simulink model "p5"  (R2020a)
settings: Solver=VariableStepAuto  StartTime=0.0  StopTime=inf  RelTol=1e-3
undefined symbols (not defined in the file): serial
libraries: instrumentlib x2
settings Model: Creator=escob  LastModifiedBy=escob

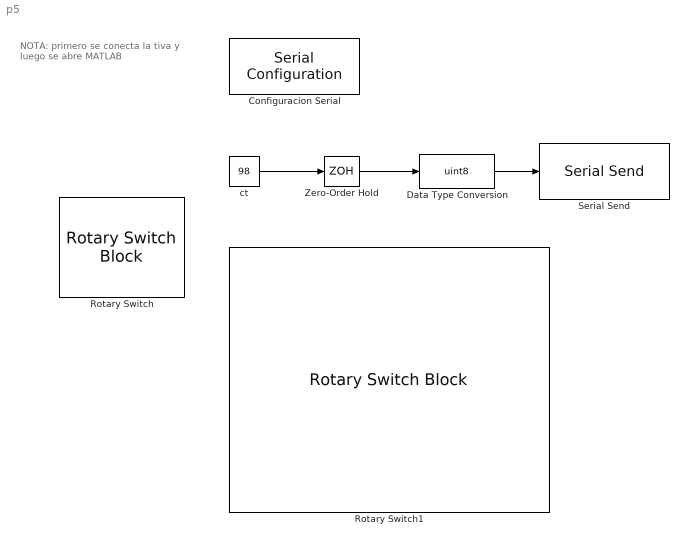
== system p5 ==
  note: NOTA: primero se conecta la tiva y
      | luego se abre MATLAB
  Configuracion Serial : instrumentlib/Serial Configuration  Priority=-200000  ComPortMenu=COM1  ComPort=COM1  ObjConstructor=serial('COM1');  BaudRate=9600  DataBits=8  Parity=none  StopBits=1  FlowControl=none  Timeout=10  ByteOrder=LittleEndian
  "Data Type Conversion " : DataTypeConversion  OutDataTypeStr=uint8
  Rotary Switch : RotarySwitchBlock
      settings: Values={{'R', 'G', 'B'}, [0 1 2]}
  Rotary Switch1 : RotarySwitchBlock
      settings: Values={{'0%', '5%', '10%', '15%', '20%', '25%', '30%', '35%', '40%', '45%', '50%', '55%', '60%', '65%', '70%', '75%', '80%', '85%', '90%', '95%', '100%', 'R', 'G', 'B'}, [1 5 10 15 20 25 30 35 40 45 50 55 60 65 70 75 80 85 90 95 100 114 103 98]}
  Serial Send : instrumentlib/Serial Send  ComPortMenu=COM1  ComPort=COM1  ObjConstructor=serial('COM1');  Terminator=<none>  EnableBlockingMode=on
  Zero-Order Hold : ZeroOrderHold  SampleTime=0.5
  ct : Constant  Value=98
  wires:
  "Data Type Conversion "/1 -> Serial Send/1
  Zero-Order Hold/1 -> "Data Type Conversion "/1
  ct/1 -> Zero-Order Hold/1
